simulink model "mass_spring_damper_Kalman"  (R2019b)
settings: Solver=FixedStepAuto  StartTime=0.0  StopTime=50  FixedStep=0.01  RelTol=1e-3
values from neighbouring files (symbols this model uses):
  A = [0.969169519504925  -0.246386829627017;  0.049277365925403  0.993808202467626]    [DMDc_MW.m]    (also in DMDc_param_sweep.m = real(A); EKF_msd_estimator.m = [0, 1; -k/m, -b/m]; HAVOK.m = AB(:,1:q*m); HAVOK_param_sweep.m = real(A))
  B = [0.049277365925403; 0.001238359506475]    [DMDc_MW.m]    (also in DMDc_param_sweep.m = AB(:,(q*m+1):end); EKF_estimator.m = zeros(nx,1); EKF_msd_estimator.m = [0; 1/m]; HAVOK.m = AB(:,(q*m+1):end))
  C = [0 1]    [DMDc_MW.m]    (also in EKF_estimator.m = eye(6); EKF_msd_estimator.m = [1, 0]; KF_estimator.m = [1, 0]; LS.m)
  D = 0    [DMDc_MW.m]    (also in DMDc_param_sweep.m = (q-1)*Ts; EKF_estimator.m = m*L*L*(M+m*(1-Cx^2)); EKF_msd_estimator.m; HAVOK.m = 3.99)
  P0 = 0.01*eye(nx)    [EKF_estimator.m]    (also in EKF_msd_estimator.m = [0.1, 0.1; 0.1, 0.1]; KF_estimator.m = [0, 0; 0, 0]; cart_pend_EKF_script.m = 0.1*eye(nx); cart_pend_EKF_setup.m = 0.1*eye(nx))
  Q = 0.01*eye(nx)    [EKF_estimator.m]    (also in EKF_msd_estimator.m = 0.00000001*eye(nx); KF_estimator.m = B*(sigma_a^2)*B'; cart_pend_EKF_script.m = 0.0000001*eye(nx); cart_pend_EKF_setup.m = diag([0; 0.00001; 0; 0.00001; 0.00001; 0.00001; 0.00001; 0.0)
  R = 0.0001*eye(ny)    [EKF_estimator.m]    (also in EKF_msd_estimator.m = 0.01*eye(ny); KF_estimator.m = 0.01; cart_pend_EKF_script.m = 0.01*eye(ny); cart_pend_EKF_setup.m = 0.001*eye(ny))
  Ts = 0.05    [DMDc_MW.m]    (also in DMDc_param_sweep.m = t(2)-t(1); EKF_msd_estimator.m = 0.01; HAVOK.m = t(2)-t(1); HAVOK_param_sweep.m = t(2)-t(1))
  x0 = [0; 0; 0; 0; 0; 1]    [EKF_estimator.m]    (also in EKF_msd_estimator.m = [0; 0]; HAVOK.m = [0.5; 0]; KF_estimator.m = [0; 0]; Linear_regression_state_estimator.m = [0;0;0;0])
settings Model: Creator=Murray  LastModifiedBy=Murray

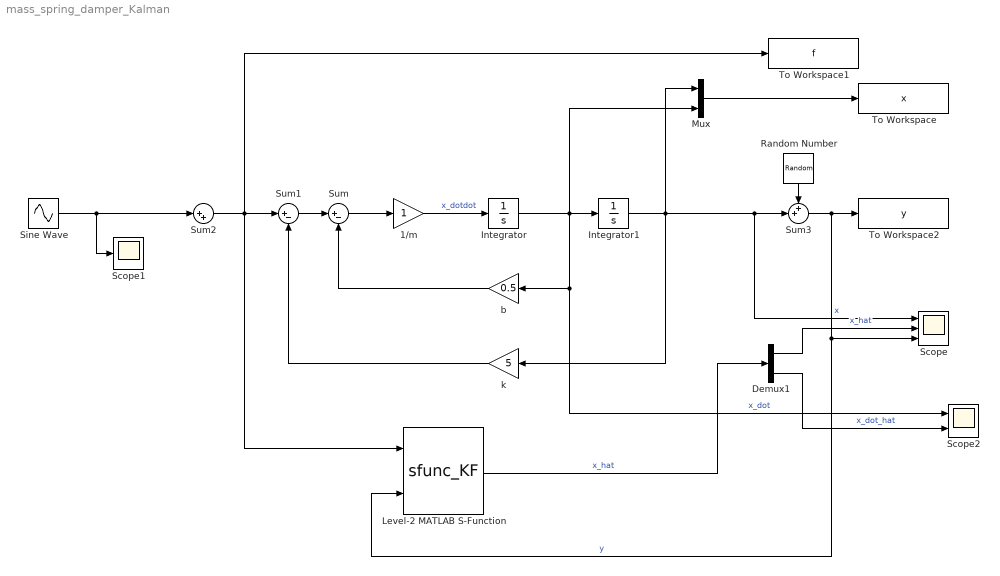
== system mass_spring_damper_Kalman ==
  1/m : Gain
  Demux1 : Demux  Outputs=2
  Integrator : Integrator
  Integrator1 : Integrator
  Level-2 MATLAB S-Function : M-S-Function  FunctionName=sfunc_KF  Parameters=A,B,C,D,Ts,Q,R,x0,P0
      mask Display:
      | port_label('input', 1, 'u')
      | port_label('input', 2, 'y')
      | port_label('output', 1, 'x_hat')
  Mux : Mux  Inputs=2
  Random Number : RandomNumber  Variance=0.08  SampleTime=0.01
  Scope : Scope  NumInputPorts=3
  Scope1 : Scope
  Scope2 : Scope  NumInputPorts=2
  Sine Wave : Sin  Bias=2  Frequency=pi/2  SampleTime=0
  Sum : Sum  Inputs=|+-
  Sum1 : Sum  Inputs=|+-
  Sum2 : Sum  Inputs=|++
  Sum3 : Sum  Inputs=++|
  To Workspace : ToWorkspace  VariableName=x  SaveFormat=Timeseries  SampleTime=-1
  To Workspace1 : ToWorkspace  VariableName=f  SaveFormat=Timeseries  SampleTime=-1
  To Workspace2 : ToWorkspace  VariableName=y  SaveFormat=Timeseries  SampleTime=-1
  b : Gain  Gain=0.5
  k : Gain  Gain=5
  wires:
  1/m/1 -> Integrator/1  "x_dotdot"
  Sum/1 -> 1/m/1
  Integrator/1 -> Scope2/1, b/1, Mux/2, Integrator1/1  "x_dot"
  b/1 -> Sum/2
  Sum1/1 -> Sum/1
  Integrator1/1 -> Mux/1, k/1, Scope/1, Sum3/2  "x"
  Sum2/1 -> Level-2 MATLAB S-Function/1, To Workspace1/1, Sum1/1
  Sine Wave/1 -> Scope1/1, Sum2/1
  k/1 -> Sum1/2
  Random Number/1 -> Sum3/1
  Mux/1 -> To Workspace/1
  Sum3/1 -> To Workspace2/1, Level-2 MATLAB S-Function/2, Scope/3  "y"
  Level-2 MATLAB S-Function/1 -> Demux1/1  "x_hat"
  Demux1/1 -> Scope/2  "x_hat"
  Demux1/2 -> Scope2/2  "x_dot_hat"
